simulink model "TestBench_DSD"  (R2021a)
settings: Solver=VariableStepAuto  StartTime=0.0  StopTime=0.05  FixedStep=1e-10  MaxStep=1e-4  RelTol=1e-3
PreLoadFcn:
  | clear;
  | dead_time= 5e-7;
  | T_sample = 1e-7;
  | f_pwm= 8e3;
  | f_el=200;
  | amplitude=0.1;
  | U_dc=800;
  | Iq_soll=200;
  | 
  | load('busdef.mat')
  | 
  | %**** Controller ****
  | L_filter = 70e-6;
  | R_losses = 1.74e-3;
  | PGain = L_filter*0.05*2*pi;
  | IGain = R_losses*0.05*2*pi;
  | 
  | %**** Deadtime Correction ****
  | Rds_on_module = 0.045/15;
  | 
  | %**** Filter ****
  | FilterQuality = 0.7071
InitFcn:
  | %%PGain = (L_filter*0.09*2*pi*f_pwm-R_losses)*0.45;
  | %%IGain = PGain*50/1.2; %% 25 = Period for ringing with too hight PGain
  | 
  | %%PGain = L_filter/(2*(1.5/f_pwm));
  | %%IGain  = PGain*R_losses/L_filter;
undefined symbols (not defined in the file): DiscIntNeverNeededParam, haltPwmSi, haltPwmSic, I_abc_sampled
libraries: nesl_utility x18, simulink x17, fl_lib x15, ee_lib x5, spsFirstOrderFilterLib x3, eeTransforms x2, cstextras x1, spsRMSLib x1, simulink_extras x1, spspowerguiLib x1
(part 1 of 3)
settings Model: Creator=Z634594  LastModifiedBy=Z634594
settings SolverCC: ZeroCrossAlgorithm=Adaptive  AlgebraicLoopSolver=TrustRegion
settings DataIOCC: ReturnWorkspaceOutputs=off
settings DebuggingCC: MergeDetectMultiDrivingBlocksExec=none  SFMachineParentedDataDiag=warning  ArithmeticOperatorsInVariantConditions=warning
settings SFSimCC: SimUseLocalCustomCode=off  CustomCodeUndefinedFunction=UseInterfaceOnly
settings RTWCC: RTWUseLocalCustomCode=off
settings CodeAppCC: StateflowObjectComments=on

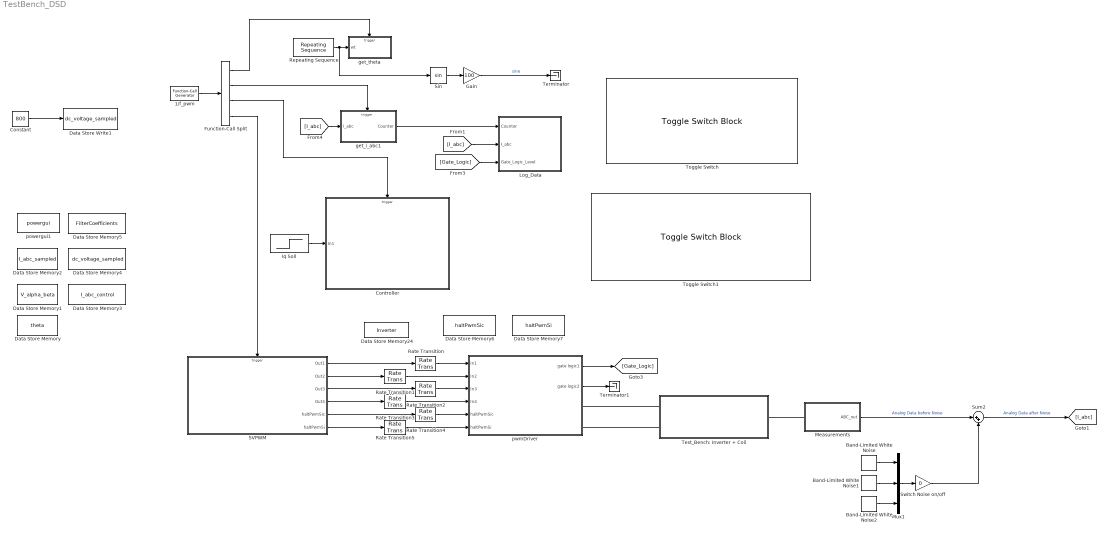
== system TestBench_DSD ==
  1/f_pwm : simulink/Ports & Subsystems/Function-Call Generator  sample_time=1/f_pwm  numberOfIterations=1  DisallowWideOutput=off
  Band-Limited White Noise : simulink/Sources/Band-Limited White Noise  Cov=[0.0004]  Ts=pi/2*1e-6  seed=[40000]
  Band-Limited White Noise1 : simulink/Sources/Band-Limited White Noise  Cov=[0.0004]  Ts=pi/2*1e-6  seed=[35000]
  Band-Limited White Noise2 : simulink/Sources/Band-Limited White Noise  Cov=[0.0004]  Ts=pi/2*1e-6  seed=[30000]
  Constant : Constant  Value=800
  Controller : Subsystem  TreatAsAtomicUnit=on
  Data Store Memory : DataStoreMemory  DataStoreName=theta  ReadBeforeWriteMsg=warning  WriteAfterWriteMsg=warning  WriteAfterReadMsg=warning  ShowAdditionalParam=off
  Data Store Memory1 : DataStoreMemory  DataStoreName=V_alpha_beta  ReadBeforeWriteMsg=warning  WriteAfterWriteMsg=warning  WriteAfterReadMsg=warning  InitialValue=[0 0]  ShowAdditionalParam=off
  Data Store Memory2 : DataStoreMemory  DataStoreName=I_abc_sampled  ReadBeforeWriteMsg=warning  WriteAfterWriteMsg=warning  WriteAfterReadMsg=warning  InitialValue=[0 0 0]  ShowAdditionalParam=off
  Data Store Memory24 : DataStoreMemory  DataStoreName=Inverter  ReadBeforeWriteMsg=warning  WriteAfterWriteMsg=warning  WriteAfterReadMsg=warning  InitialValue=Device_MATLABStruct  ShowAdditionalParam=off  OutDataTypeStr=Bus: Device
  Data Store Memory3 : DataStoreMemory  DataStoreName=I_abc_control  ReadBeforeWriteMsg=warning  WriteAfterWriteMsg=warning  WriteAfterReadMsg=warning  InitialValue=[0 0 0]  ShowAdditionalParam=off
  Data Store Memory4 : DataStoreMemory  DataStoreName=dc_voltage_sampled  ReadBeforeWriteMsg=warning  WriteAfterWriteMsg=warning  WriteAfterReadMsg=warning  InitialValue=U_dc  ShowAdditionalParam=off
  Data Store Memory5 : DataStoreMemory  DataStoreName=FilterCoefficients  ReadBeforeWriteMsg=warning  WriteAfterWriteMsg=warning  WriteAfterReadMsg=warning  InitialValue=[1 0 0 0 0]  ShowAdditionalParam=off
  Data Store Memory6 : DataStoreMemory  DataStoreName=haltPwmSic  ReadBeforeWriteMsg=warning  WriteAfterWriteMsg=warning  WriteAfterReadMsg=warning  InitialValue=[1 1 1]  ShowAdditionalParam=off
  Data Store Memory7 : DataStoreMemory  DataStoreName=haltPwmSi  ReadBeforeWriteMsg=warning  WriteAfterWriteMsg=warning  WriteAfterReadMsg=warning  InitialValue=[0 0 0]  ShowAdditionalParam=off
  Data Store Write1 : DataStoreWrite  DataStoreName=dc_voltage_sampled  IndexOptions=Index vector (dialog)  Indices=1  OutputSizes=1
  Function-Call Split : FunctionCallSplit  IconShape=distinctive  NumOutputPorts=4  OutputPortLayout=default
  Gain : Gain  Gain=100
  Iq Soll : Step  Time=2/f_pwm  After=Iq_soll  SampleTime=0
  Log_Data : Subsystem
  Measurements : Subsystem
  Mux1 : Mux  Inputs=3
  Rate Transition{,1..5} (6 alike) : RateTransition
  Repeating Sequence : simulink/Sources/Repeating Sequence  rep_seq_t=[0 1/f_el]  rep_seq_y=[0 2*pi]
  SVPWM : Subsystem
  Sin : Trigonometry
  Sum2 : Sum  Inputs=|++
  Switch Noise on/off : Gain  Gain=0
  Terminator : Terminator
  Terminator1 : Terminator
  Test_Bench: Inverter + Coil : Subsystem
  Toggle Switch : ToggleSwitchBlock
      settings: Values={{'Off', 'On'}, [0 1]}
  Toggle Switch1 : ToggleSwitchBlock
      settings: Values={{'Off', 'On'}, [0 1]}
  get_i_abc1 : Subsystem  TreatAsAtomicUnit=on
  get_theta : Subsystem  TreatAsAtomicUnit=on
  powergui1 : spspowerguiLib/powergui  Priority=1  SimulationMode=Continuous  SampleTime=1e-9  frequency=60  Iterations=50  frequencyindice=0  Pbase=100e6  ErrMax=1e-4  UnitsV=kV  UnitsW=MW  buscounter=0  FunctionMessages=off  echomessages=off  EnableUseOfTLC=off  CurrentSourceSwitches=off  DisableSnubberDevices=off  DisableRonSwitches=off  DisableVfSwitches=off  DisplayEquations=off  AutomaticDiscreteSolvers=off  SolverType=Tustin/Backward Euler (TBE)  Interpol=off  ExternalGateDelay=off  methode=off  Ts=100  x0status=blocks  SPID=on  SwTol=0  HookPort=off  NonlinearTolerance=1e-4  nMaxIteration=100  ContinueOnMaxIteration=off  RestoreLinks=warning  ResistiveCurrentMeasurement=off  Frange=[0:2:500]  Ylog=off  Xlog=on  ShowGrid=off  save=off  variable=ZData  structure=logsout  ZoomFFT=off  StartTime=0.01  cycles=10  DisplayStyle=1  fundamental=200  FreqAxis=off  MaxFrequency=10000  frequencyindicesteady=1  RmsSteady=1  display=off
  pwmDriver : Subsystem
  wires:
  Repeating Sequence/1 -> Sin/1, get_theta/1(wt)
  [I_abc] -> Log_Data/2(I_abc)
  [Gate_Logic] -> Log_Data/3(Gate_Logic_Level)
  Sum2/1 -> [I_abc]  "Analog Data after Noise"
  Band-Limited White Noise1/1 -> Mux1/2
  Band-Limited White Noise/1 -> Mux1/1
  Band-Limited White Noise2/1 -> Mux1/3
  Mux1/1 -> Switch Noise on/off/1
  Measurements/1(ABC_out) -> Sum2/1  "Analog Data before Noise"
  Switch Noise on/off/1 -> Sum2/2
  Constant/1 -> Data Store Write1/1
  get_i_abc1/1(Counter) -> Log_Data/1(Counter)
  pwmDriver/1(gate logic1) -> [Gate_Logic]
  [I_abc] -> get_i_abc1/1(I_abc)
  1/f_pwm/1 -> Function-Call Split/1
  Function-Call Split/1 -> get_theta/Trigger
  Function-Call Split/2 -> get_i_abc1/Trigger
  Function-Call Split/3 -> Controller/Trigger
  Iq Soll/1 -> Controller/1(In1)
  Function-Call Split/4 -> SVPWM/Trigger
  SVPWM/4(Out4) -> Rate Transition3/1
  SVPWM/3(Out3) -> Rate Transition2/1
  SVPWM/2(Out2) -> Rate Transition1/1
  SVPWM/1(Out1) -> Rate Transition/1
  Rate Transition/1 -> pwmDriver/1(In1)
  Rate Transition1/1 -> pwmDriver/2(In2)
  Rate Transition2/1 -> pwmDriver/3(In3)
  Rate Transition3/1 -> pwmDriver/4(In4)
  Rate Transition4/1 -> pwmDriver/5(haltPwmSic)
  SVPWM/5(haltPwmSic) -> Rate Transition4/1
  SVPWM/6(haltPwmSi) -> Rate Transition5/1
  Rate Transition5/1 -> pwmDriver/6(haltPwmSi)
  Sin/1 -> Gain/1
  Gain/1 -> Terminator/1  "sine"
  pwmDriver/2(gate logic2) -> Terminator1/1
  connections:
  Test_Bench: Inverter + Coil/LConn1 -- pwmDriver/RConn1
  Measurements/LConn1 -- Test_Bench: Inverter + Coil/RConn1
  Test_Bench: Inverter + Coil/LConn2 -- pwmDriver/RConn2

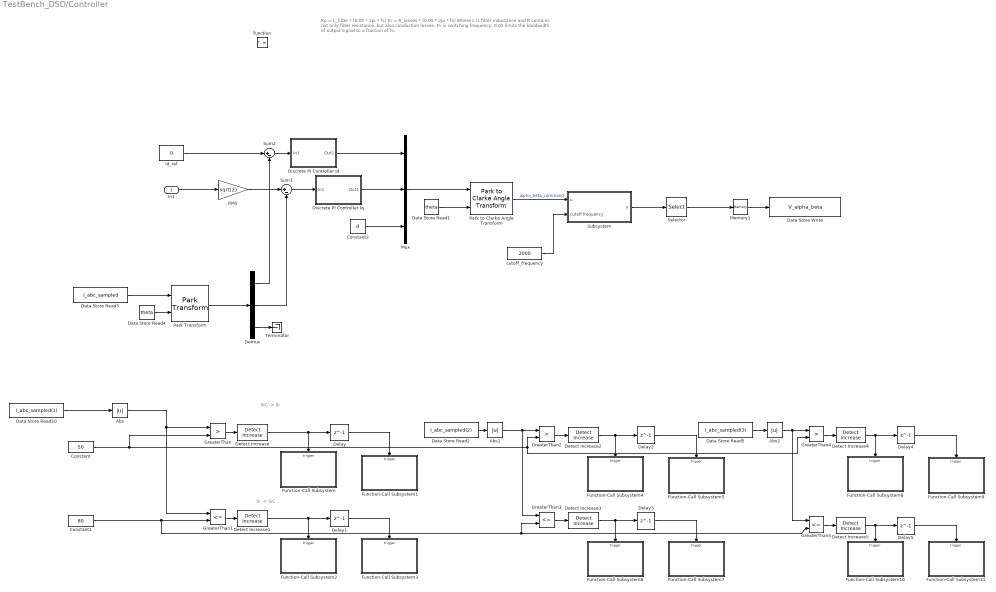
== system TestBench_DSD/Controller ==
  note: Kp = L_filter * (0.05 * 2pi * fs)
      |
      | Ki = R_losses * (0.05 * 2pi * fs)
      |
      | Where L is filter inductance and R contains not only filter resistance, but also conduction losses.
      | Fs is switching frequency.
      | 0.05 limits the bandwidth of output signal to a fraction of fs.
  note: Si -> SiC
  note: SiC -> Si
  In1 : Inport
  function : TriggerPort  TriggerType=function-call  VariantControl=Variant
  Abs : Abs
  Abs1 : Abs
  Abs2 : Abs
  Constant : Constant  Value=50
  Constant1 : Constant  Value=80
  Constant2 : Constant  Value=0
  Data Store Read1 : DataStoreRead  DataStoreName=theta  IndexOptions=Index vector (dialog)  Indices=1  OutputSizes=1
  Data Store Read10 : DataStoreRead  DataStoreName=I_abc_sampled  DataStoreElements=I_abc_sampled(1)  IndexOptions=Index vector (dialog)  Indices=1  OutputSizes=1
  Data Store Read2 : DataStoreRead  DataStoreName=I_abc_sampled  DataStoreElements=I_abc_sampled(2)  IndexOptions=Index vector (dialog)  Indices=1  OutputSizes=1
  Data Store Read3 : DataStoreRead  DataStoreName=I_abc_sampled  IndexOptions=Index vector (dialog)  Indices=1  OutputSizes=1
  Data Store Read4 : DataStoreRead  DataStoreName=theta  IndexOptions=Index vector (dialog)  Indices=1  OutputSizes=1
  Data Store Read5 : DataStoreRead  DataStoreName=I_abc_sampled  DataStoreElements=I_abc_sampled(3)  IndexOptions=Index vector (dialog)  Indices=1  OutputSizes=1
  Data Store Write : DataStoreWrite  DataStoreName=V_alpha_beta  IndexOptions=Index vector (dialog)  Indices=1  OutputSizes=1
  Delay{,1..5} (6 alike) : Delay  DelayLength=1
  Demux : Demux  Outputs=3
  Detect Increase{,1..5} (6 alike) : simulink/Logic and Bit Operations/Detect Increase  vinit=0.0  OutDataTypeStr=boolean
  Discrete PI Controller Id : Subsystem
  Discrete PI Controller Iq : Subsystem
  Function-Call Subsystem : Subsystem  TreatAsAtomicUnit=on
  Function-Call Subsystem1 : Subsystem  TreatAsAtomicUnit=on
  Function-Call Subsystem10 : Subsystem  TreatAsAtomicUnit=on
  Function-Call Subsystem11 : Subsystem  TreatAsAtomicUnit=on
  Function-Call Subsystem2 : Subsystem  TreatAsAtomicUnit=on
  Function-Call Subsystem3 : Subsystem  TreatAsAtomicUnit=on
  Function-Call Subsystem4 : Subsystem  TreatAsAtomicUnit=on
  Function-Call Subsystem5 : Subsystem  TreatAsAtomicUnit=on
  Function-Call Subsystem6 : Subsystem  TreatAsAtomicUnit=on
  Function-Call Subsystem7 : Subsystem  TreatAsAtomicUnit=on
  Function-Call Subsystem8 : Subsystem  TreatAsAtomicUnit=on
  Function-Call Subsystem9 : Subsystem  TreatAsAtomicUnit=on
  GreaterThan : RelationalOperator  Operator=>  OutDataTypeStr=boolean  RndMeth=Simplest
  GreaterThan1 : RelationalOperator  Operator=<=  OutDataTypeStr=boolean  RndMeth=Simplest
  GreaterThan2 : RelationalOperator  Operator=>  OutDataTypeStr=boolean  RndMeth=Simplest
  GreaterThan3 : RelationalOperator  Operator=<=  OutDataTypeStr=boolean  RndMeth=Simplest
  GreaterThan4 : RelationalOperator  Operator=>  OutDataTypeStr=boolean  RndMeth=Simplest
  GreaterThan5 : RelationalOperator  Operator=<=  OutDataTypeStr=boolean  RndMeth=Simplest
  Id_ref : Constant  Value=0
  Memory1 : Memory  InheritSampleTime=on  LinearizeAsDelay=on
  Mux : Mux  Inputs=3
  Park Transform : eeTransforms/Park Transform  AxisAlignment=Q-axis  PowerInvariant=off
  Park to Clarke Angle Transform : eeTransforms/Park to Clarke Angle Transform  AxisAlignment=Q-axis
      settings: SourceProductBaseCode=PS
  RMS : Gain  Gain=sqrt(2)
  Selector : Selector  InputPortWidth=3  IndexOptions=Index vector (dialog)  Indices=[1 2]  OutputSizes=1
  Subsystem : Subsystem
  Sum1 : Sum  Inputs=|+-
  Sum2 : Sum  Inputs=|+-
  Terminator : Terminator
  cutoff_frequency : Constant  Value=2000
  wires:
  Demux/1 -> Sum2/2
  Mux/1 -> Park to Clarke Angle Transform/1
  Demux/3 -> Terminator/1
  Demux/2 -> Sum1/2
  Constant2/1 -> Mux/3
  Sum2/1 -> Discrete PI Controller Id/1(In1)
  Sum1/1 -> Discrete PI Controller Iq/1(In1)
  Discrete PI Controller Iq/1(Out1) -> Mux/2
  Data Store Read3/1 -> Park Transform/1
  Data Store Read4/1 -> Park Transform/2
  Data Store Read1/1 -> Park to Clarke Angle Transform/2
  Memory1/1 -> Data Store Write/1
  Discrete PI Controller Id/1(Out1) -> Mux/1
  Park Transform/1 -> Demux/1
  Selector/1 -> Memory1/1
  Id_ref/1 -> Sum2/1
  In1/1 -> RMS/1
  RMS/1 -> Sum1/1
  cutoff_frequency/1 -> Subsystem/2(cutoff frequency)
  Park to Clarke Angle Transform/1 -> Subsystem/1(u)  "alpha_beta_command"
  Subsystem/1(y) -> Selector/1
  Delay1/1 -> Function-Call Subsystem3/Trigger
  Delay/1 -> Function-Call Subsystem1/Trigger
  Delay2/1 -> Function-Call Subsystem5/Trigger
  Delay5/1 -> Function-Call Subsystem11/Trigger
  Delay4/1 -> Function-Call Subsystem9/Trigger
  GreaterThan1/1 -> Detect Increase1/1
  Delay3/1 -> Function-Call Subsystem7/Trigger
  GreaterThan/1 -> Detect Increase/1
  Data Store Read10/1 -> Abs/1
  Abs/1 -> GreaterThan1/1, GreaterThan/1
  Data Store Read2/1 -> Abs1/1
  Abs1/1 -> GreaterThan3/1, GreaterThan2/1
  GreaterThan2/1 -> Detect Increase2/1
  GreaterThan3/1 -> Detect Increase3/1
  Data Store Read5/1 -> Abs2/1
  Abs2/1 -> GreaterThan5/1, GreaterThan4/1
  Constant/1 -> GreaterThan/2, GreaterThan4/2, GreaterThan2/2
  Constant1/1 -> GreaterThan5/2, GreaterThan3/2, GreaterThan1/2
  Detect Increase/1 -> Delay/1, Function-Call Subsystem/Trigger
  Detect Increase1/1 -> Delay1/1, Function-Call Subsystem2/Trigger
  Detect Increase2/1 -> Function-Call Subsystem4/Trigger, Delay2/1
  Detect Increase3/1 -> Function-Call Subsystem6/Trigger, Delay3/1
  GreaterThan4/1 -> Detect Increase4/1
  Detect Increase4/1 -> Function-Call Subsystem8/Trigger, Delay4/1
  GreaterThan5/1 -> Detect Increase5/1
  Detect Increase5/1 -> Function-Call Subsystem10/Trigger, Delay5/1

== system TestBench_DSD/Log_Data ==
  Counter : Inport
  I_abc : Inport  Port=2
  Gate_Logic_Level : Inport  Port=3
  Data Store Read1 : DataStoreRead  DataStoreName=I_abc_sampled  IndexOptions=Index vector (dialog)  Indices=1  OutputSizes=1
  Data Store Read2 : DataStoreRead  DataStoreName=I_abc_control  IndexOptions=Index vector (dialog)  Indices=1  OutputSizes=1
  Delay : Delay  DelayLength=1  SampleTime=T_sample
  Gain : Gain  Gain=50
  Logical Operator : Logic  Operator=XOR  AllPortsSameDT=off  OutDataTypeStr=boolean
  Product : Product
  Scope1 : Scope  NumInputPorts=3
  Scope6 : Scope  NumInputPorts=5
  wires:
  Delay/1 -> Scope1/2, Logical Operator/1
  Data Store Read1/1 -> Product/2, Scope6/1
  Counter/1 -> Scope1/1, Logical Operator/2, Delay/1
  Product/1 -> Scope6/3
  Logical Operator/1 -> Scope1/3, Product/1
  Gain/1 -> Scope6/4
  I_abc/1 -> Scope6/2
  Gate_Logic_Level/1 -> Gain/1
  Data Store Read2/1 -> Scope6/5

== system TestBench_DSD/Measurements ==
  First-Order Filter : spsFirstOrderFilterLib/First-Order Filter  FilterType=Lowpass  Tc=25e-6  Ts=0  Initialize=off  Vac_Init=[0, 0, 60]  Vdc_Init=0  PlotResponse=off  FreqRange="[0,  200,  1]"
  PS-Simulink Converter1 : nesl_utility/PS-Simulink Converter  PhysicalDomain=network_engine_domain  SubClassName=ps_output  LeftPortType=input  RightPortType=output  PseudoPeriodic=off  Frequencies=[]  Unit=1  AffineConversion=off
      settings: SourceProductBaseCode=PW,SS
  RMS : spsRMSLib/RMS  TrueRMS=on  Freq=f_el  RMSInit=0  Ts=0
  Terminator : Terminator
  Terminator1 : Terminator
  ABC_in : PMIOPort  Side=Left
  ABC_out : Outport  VectorParamsAs1DForOutWhenUnconnected=off
  wires:
  PS-Simulink Converter1/1 -> RMS/1, First-Order Filter/1, ABC_out/1
  RMS/1 -> Terminator/1  "rmsCurrent3Phase"
  First-Order Filter/1 -> Terminator1/1  "phaseCurrent3Phase"
  connections:
  PS-Simulink Converter1/LConn1 -- ABC_in/RConn1

== system TestBench_DSD/SVPWM ==
  function : TriggerPort  TriggerType=function-call  VariantControl=(inherit)
  Data Store Read : DataStoreRead  DataStoreName=V_alpha_beta  IndexOptions=Index vector (dialog)  Indices=1  OutputSizes=1
  Data Store Read1 : DataStoreRead  DataStoreName=I_abc_sampled  IndexOptions=Index vector (dialog)  Indices=1  OutputSizes=1
  Data Store Read2 : DataStoreRead  DataStoreName=dc_voltage_sampled  IndexOptions=Index vector (dialog)  Indices=1  OutputSizes=1
  Data Store Read5 : DataStoreRead  DataStoreName=dc_voltage_sampled  IndexOptions=Index vector (dialog)  Indices=1  OutputSizes=1
  Demux : Demux  Outputs=2
  Divide : Product  Inputs=*/
  Gate_Signal_Voltage1 : Subsystem
  Model : ModelReference  ModelNameDialog=sort_dutycycles.slx  SimulationMode=Normal  ModelReferenceVersion=1.5
  SVPWM : Subsystem
  Terminator : Terminator
  Out1 : Outport
  Out2 : Outport  Port=2
  Out3 : Outport  Port=3
  Out4 : Outport  Port=4
  haltPwmSic : Outport  Port=5
  haltPwmSi : Outport  Port=6
  wires:
  Divide/1 -> Demux/1
  Data Store Read5/1 -> Divide/2
  SVPWM/1(Sector Number) -> Model/1
  SVPWM/2(Ta Tb T0 normalized) -> Model/2
  Data Store Read/1 -> Divide/1
  Demux/2 -> SVPWM/2(U_angle)
  Model/2 -> Terminator/1
  Demux/1 -> SVPWM/1(U_mag)
  Model/1 -> Gate_Signal_Voltage1/1(dutycycles)  "Duty Cycles Rearranged"
  Data Store Read1/1 -> Gate_Signal_Voltage1/2(phaseCurrent)
  Gate_Signal_Voltage1/2(Out2) -> Out2/1
  Gate_Signal_Voltage1/4(Out4) -> Out4/1
  Gate_Signal_Voltage1/3(Out3) -> Out3/1
  Gate_Signal_Voltage1/1(Out1) -> Out1/1
  Gate_Signal_Voltage1/5(haltPwmSic) -> haltPwmSic/1
  Gate_Signal_Voltage1/6(haltPwmSi) -> haltPwmSi/1
  Data Store Read2/1 -> Gate_Signal_Voltage1/3(dcLinkVoltage)

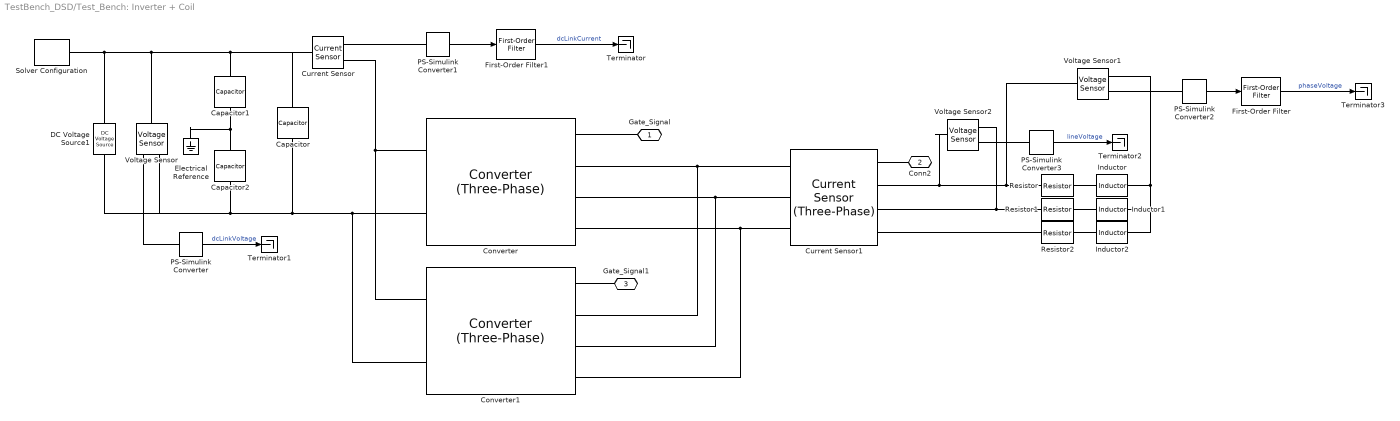
== system TestBench_DSD/Test_Bench: Inverter + Coil ==
  Capacitor : fl_lib/Electrical/Electrical Elements/Capacitor  c=550e-6 F  r=1e-6 Ohm  g=0 1/Ohm  i_specify=off  i_priority=None  i=0 A  i_nominal_specify=off  i_nominal_unit=A  i_nominal_value=1  v_specify=off  v_priority=None  v=0 V  v_nominal_specify=off  v_nominal_unit=V  v_nominal_value=1  vc_specify=on  vc_priority=High  vc=U_dc V  vc_nominal_specify=off  vc_nominal_unit=V  vc_nominal_value=1
  Capacitor1 : fl_lib/Electrical/Electrical Elements/Capacitor  c=100e-9 F  r=1e-6 Ohm  g=0 1/Ohm  i_specify=off  i_priority=None  i=0 A  i_nominal_specify=off  i_nominal_unit=A  i_nominal_value=1  v_specify=off  v_priority=None  v=0 V  v_nominal_specify=off  v_nominal_unit=V  v_nominal_value=1  vc_specify=on  vc_priority=High  vc=U_dc/2 V  vc_nominal_specify=off  vc_nominal_unit=V  vc_nominal_value=1
  Capacitor2 : fl_lib/Electrical/Electrical Elements/Capacitor  c=100e-9 F  r=1e-6 Ohm  g=0 1/Ohm  i_specify=off  i_priority=None  i=0 A  i_nominal_specify=off  i_nominal_unit=A  i_nominal_value=1  v_specify=off  v_priority=None  v=0 V  v_nominal_specify=off  v_nominal_unit=V  v_nominal_value=1  vc_specify=on  vc_priority=High  vc=U_dc/2 V  vc_nominal_specify=off  vc_nominal_unit=V  vc_nominal_value=1
  Converter : ee_lib/Semiconductors & Converters/Converters/Converter (Three-Phase)  device_type=ee.enum.converters.switchingdevice.mosfet  Vf=0.8 V  Ron=0.001 Ohm  Rds=Rds_on_module Ohm  Goff=1e-9 1/Ohm  Vth=4 V  Vgt=1 V  Vgt_off=-1 V  Ih=1 A  diode_param=ee.enum.converters.protectiondiode.nodynamics  diode_Vf=2 V  diode_Ron=Rds_on_module Ohm  diode_Goff=1e-9 1/Ohm  diode_C=50 nF  diode_iRM=-235 A  diode_iF=300 A  diode_idot=-50 A/us  diode_trr_param=ee.enum.converters.diodetrr.trr_factor  diode_trr_factor=3  diode_trr=15 us  diode_Qrr=1.5e+3 s*uA  snubber_type=ee.enum.converters.snubber.exclude  Rs=0.01 Ohm  Cs=1e-6 F
      settings: SourceProductBaseCode=PS  InternalSimscapePortConfiguration="{\"Bottom\":[],\"Left\":[{\"id\":\"G\",\"label\":\"G\",\"type\":\"foundation.electrical.twelve_phase\"},{\"id\":\"a\",\"label\":\"a\",\"type\":\"foundation.electrical.electrical\"},{\"id\":\"b\",\"label\":\"b\",\"type\":\"foundation.electrical.electrical\"},{\"id\":\"c\",\"label\":\"c\",\"type\":\"foundation.electrical.electrical\"}],\"Right\":[{\"id\":\"p\",\"label\":\"+\",\"type\":\"foundation.electrical.electrical\"},{\"id\":\"n\",\"label\":\"-\",\"type\":\"foundation.electrical.electrical\"}],\"Top\":[]}"
  Converter1 : ee_lib/Semiconductors & Converters/Converters/Converter (Three-Phase)  device_type=ee.enum.converters.switchingdevice.igbt  Vf=0.8 V  Ron=0.001 Ohm  Rds=Rds_on_module Ohm  Goff=1e-9 1/Ohm  Vth=4 V  Vgt=1 V  Vgt_off=-1 V  Ih=1 A  diode_param=ee.enum.converters.protectiondiode.nodynamics  diode_Vf=0.8 V  diode_Ron=0.001 Ohm  diode_Goff=1e-9 1/Ohm  diode_C=50 nF  diode_iRM=-235 A  diode_iF=300 A  diode_idot=-50 A/us  diode_trr_param=ee.enum.converters.diodetrr.trr_factor  diode_trr_factor=3  diode_trr=15 us  diode_Qrr=1.5e+3 s*uA  snubber_type=ee.enum.converters.snubber.exclude  Rs=0.01 Ohm  Cs=1e-6 F
      settings: SourceProductBaseCode=PS  InternalSimscapePortConfiguration="{\"Bottom\":[],\"Left\":[{\"id\":\"G\",\"label\":\"G\",\"type\":\"foundation.electrical.twelve_phase\"},{\"id\":\"a\",\"label\":\"a\",\"type\":\"foundation.electrical.electrical\"},{\"id\":\"b\",\"label\":\"b\",\"type\":\"foundation.electrical.electrical\"},{\"id\":\"c\",\"label\":\"c\",\"type\":\"foundation.electrical.electrical\"}],\"Right\":[{\"id\":\"p\",\"label\":\"+\",\"type\":\"foundation.electrical.electrical\"},{\"id\":\"n\",\"label\":\"-\",\"type\":\"foundation.electrical.electrical\"}],\"Top\":[]}"
  Current Sensor : fl_lib/Electrical/Electrical Sensors/Current Sensor
  Current Sensor1 : ee_lib/Sensors & Transducers/Current Sensor (Three-Phase)
      settings: InternalSimscapePortConfiguration="{\"Bottom\":[],\"Left\":[{\"id\":\"a1\",\"label\":\"a1\",\"type\":\"foundation.electrical.electrical\"},{\"id\":\"b1\",\"label\":\"b1\",\"type\":\"foundation.electrical.electrical\"},{\"id\":\"c1\",\"label\":\"c1\",\"type\":\"foundation.electrical.electrical\"}],\"Right\":[{\"id\":\"I_output\",\"label\":\"I\",\"type\":\"output\"},{\"id\":\"a2\",\"label\":\"a2\",\"type\":\"foundation.electrical.electrical\"},{\"id\":\"b2\",\"label\":\"b2\",\"type\":\"foundation.electrical.electrical\"},{\"id\":\"c2\",\"label\":\"c2\",\"type\":\"foundation.electrical.electrical\"}],\"Top\":[]}"
  DC Voltage Source1 : fl_lib/Electrical/Electrical Sources/DC Voltage Source  v0=U_dc V
  Electrical Reference : fl_lib/Electrical/Electrical Elements/Electrical Reference
  First-Order Filter : spsFirstOrderFilterLib/First-Order Filter  FilterType=Lowpass  Tc=250e-6  Ts=0  Initialize=off  Vac_Init=[0, 0, 60]  Vdc_Init=0  PlotResponse=off  FreqRange="[0,  200,  1]"
  First-Order Filter1 : spsFirstOrderFilterLib/First-Order Filter  FilterType=Lowpass  Tc=100e-6  Ts=0  Initialize=off  Vac_Init=[0, 0, 60]  Vdc_Init=0  PlotResponse=off  FreqRange="[0,  200,  1]"
  Inductor : fl_lib/Electrical/Electrical Elements/Inductor  l=70e-6 H  r=0 Ohm  g=1e-9 1/Ohm  i_specify=off  i_priority=None  i=0 A  i_nominal_specify=off  i_nominal_unit=A  i_nominal_value=1  v_specify=off  v_priority=None  v=0 V  v_nominal_specify=off  v_nominal_unit=V  v_nominal_value=1  i_L_specify=off  i_L_priority=High  i_L=0 A  i_L_nominal_specify=off  i_L_nominal_unit=A  i_L_nominal_value=1
  Inductor1 : fl_lib/Electrical/Electrical Elements/Inductor  l=70e-6 H  r=0 Ohm  g=1e-9 1/Ohm  i_specify=off  i_priority=None  i=0 A  i_nominal_specify=off  i_nominal_unit=A  i_nominal_value=1  v_specify=off  v_priority=None  v=0 V  v_nominal_specify=off  v_nominal_unit=V  v_nominal_value=1  i_L_specify=off  i_L_priority=High  i_L=0 A  i_L_nominal_specify=off  i_L_nominal_unit=A  i_L_nominal_value=1
  Inductor2 : fl_lib/Electrical/Electrical Elements/Inductor  l=70e-6 H  r=0 Ohm  g=1e-9 1/Ohm  i_specify=off  i_priority=None  i=0 A  i_nominal_specify=off  i_nominal_unit=A  i_nominal_value=1  v_specify=off  v_priority=None  v=0 V  v_nominal_specify=off  v_nominal_unit=V  v_nominal_value=1  i_L_specify=off  i_L_priority=High  i_L=0 A  i_L_nominal_specify=off  i_L_nominal_unit=A  i_L_nominal_value=1
  PS-Simulink Converter{,1..3} (4 alike) : nesl_utility/PS-Simulink Converter  PhysicalDomain=network_engine_domain  SubClassName=ps_output  LeftPortType=input  RightPortType=output  PseudoPeriodic=off  Frequencies=[]  Unit=1  AffineConversion=off
      settings: SourceProductBaseCode=PW,SS
  Resistor : fl_lib/Electrical/Electrical Elements/Resistor  R=1.74e-3 Ohm  i_specify=off  i_priority=None  i=0 A  i_nominal_specify=off  i_nominal_unit=A  i_nominal_value=1  v_specify=off  v_priority=None  v=0 V  v_nominal_specify=off  v_nominal_unit=V  v_nominal_value=1
  Resistor1 : fl_lib/Electrical/Electrical Elements/Resistor  R=1.74e-3 Ohm  i_specify=off  i_priority=None  i=0 A  i_nominal_specify=off  i_nominal_unit=A  i_nominal_value=1  v_specify=off  v_priority=None  v=0 V  v_nominal_specify=off  v_nominal_unit=V  v_nominal_value=1
  Resistor2 : fl_lib/Electrical/Electrical Elements/Resistor  R=1.74e-3 Ohm  i_specify=off  i_priority=None  i=0 A  i_nominal_specify=off  i_nominal_unit=A  i_nominal_value=1  v_specify=off  v_priority=None  v=0 V  v_nominal_specify=off  v_nominal_unit=V  v_nominal_value=1
  Solver Configuration : nesl_utility/Solver Configuration  PhysicalDomain=network_engine_domain  SubClassName=solver  LeftPortType=input  RightPortType=generic  Tones=[]  Harmonics=[]  SimulateNoise=off  Profile=off  UseLocalSampling=off  EnableSwitchedLinearOptims=on  FrequencyDomain=off  UseCCode=off  RelTol=0.001  AbsTol=1e-06  MinStep=1e-09  ToWorkspace=off  RevertToSquareIcSolve=off  NumHomotopyIterations=100  PhasorMode=off  PhasorModeNumHarmonics=1  DoDC=off  ResidualTolerance=1e-09  UseLocalSolver=off  LocalSolverChoice=NE_BACKWARD_EULER_ADVANCER  LocalSolverSampleTime=0.001  DoFixedCost=off  MaxNonlinIter=3  MaxModeIter=2  ComputeImpulses=off  ImpulseIterations=2  LinearAlgebra=Sparse  EquationFormulation=NE_TIME_EF  DelaysMemoryBudget=1024  AutomaticFiltering=on  FilteringTimeConstant=0.001  PartitionStorageMethod=AS_NEEDED  PartitionMemoryBudget=1024  PartitionMethod=FAST
      settings: SourceProductBaseCode=PW,SS
  Terminator{,1..3} (4 alike) : Terminator
  Voltage Sensor : fl_lib/Electrical/Electrical Sensors/Voltage Sensor
  Voltage Sensor1 : fl_lib/Electrical/Electrical Sensors/Voltage Sensor
  Voltage Sensor2 : fl_lib/Electrical/Electrical Sensors/Voltage Sensor
  Gate_Signal : PMIOPort  Side=Left
  Conn2 : PMIOPort  Port=2  Side=Right
  Gate_Signal1 : PMIOPort  Port=3  Side=Left
  wires:
  First-Order Filter1/1 -> Terminator/1  "dcLinkCurrent"
  PS-Simulink Converter/1 -> Terminator1/1  "dcLinkVoltage"
  PS-Simulink Converter1/1 -> First-Order Filter1/1
  PS-Simulink Converter2/1 -> First-Order Filter/1
  PS-Simulink Converter3/1 -> Terminator2/1  "lineVoltage"
  First-Order Filter/1 -> Terminator3/1  "phaseVoltage"
  connections:
  Voltage Sensor1/RConn2 -- Inductor2/RConn1 -- Inductor1/RConn1 -- Inductor/RConn1
  Current Sensor1/LConn1 -- Converter1/LConn2 -- Converter/LConn2
  Current Sensor1/LConn2 -- Converter1/LConn3 -- Converter/LConn3
  Current Sensor1/RConn2 -- Resistor/LConn1 -- Voltage Sensor1/LConn1 -- Voltage Sensor2/LConn1
  Resistor/RConn1 -- Inductor/LConn1
  Converter/LConn1 -- Gate_Signal/RConn1
  Resistor1/RConn1 -- Inductor1/LConn1
  Current Sensor1/RConn4 -- Resistor2/LConn1
  Current Sensor1/RConn3 -- Resistor1/LConn1 -- Voltage Sensor2/RConn2
  Resistor2/RConn1 -- Inductor2/LConn1
  Current Sensor1/LConn3 -- Converter1/LConn4 -- Converter/LConn4
  Capacitor/RConn1 -- Capacitor2/RConn1 -- DC Voltage Source1/RConn1 -- Voltage Sensor/RConn2 -- Converter1/RConn2 -- Converter/RConn2
  Current Sensor/RConn2 -- Converter1/RConn1 -- Converter/RConn1
  PS-Simulink Converter/LConn1 -- Voltage Sensor/RConn1
  PS-Simulink Converter1/LConn1 -- Current Sensor/RConn1
  Voltage Sensor/LConn1 -- Capacitor1/LConn1 -- Capacitor/LConn1 -- Current Sensor/LConn1 -- DC Voltage Source1/LConn1 -- Solver Configuration/RConn1
  Conn2/RConn1 -- Current Sensor1/RConn1
  PS-Simulink Converter2/LConn1 -- Voltage Sensor1/RConn1
  PS-Simulink Converter3/LConn1 -- Voltage Sensor2/RConn1
  Capacitor2/LConn1 -- Electrical Reference/LConn1 -- Capacitor1/RConn1
  Gate_Signal1/RConn1 -- Converter1/LConn1

== system TestBench_DSD/get_i_abc1 ==
  note: Digital Biquad Filter (IIR)
      | Transposed Direct Form 2
  I_abc : Inport
  function : TriggerPort  TriggerType=function-call  VariantControl=Variant
  Counter Limited : simulink/Sources/Counter Limited  uplimit=1  tsamp=-1
  Data Store Write : DataStoreWrite  DataStoreName=I_abc_sampled  IndexOptions=Index vector (dialog)  Indices=1  OutputSizes=1
  Delay1 : Delay  DelayLength=1
  Delay3 : Delay  DelayLength=1
  Gain : Gain  Gain=0.13491016791740667
  Gain1 : Gain  Gain=-1.1429772843080923
  Gain2 : Gain  Gain=0.41279762014290533
  Gain3 : Gain  Gain=0.06745508395870334
  Gain4 : Gain  Gain=0.06745508395870334
  Scope : Scope  NumInputPorts=3
  Sum : Sum  Inputs=++-
  Sum1 : Sum  Inputs=+|-
  Sum2 : Sum  Inputs=|++
  Counter : Outport  VectorParamsAs1DForOutWhenUnconnected=off
  wires:
  Counter Limited/1 -> Counter/1
  Gain/1 -> Sum/1
  Gain1/1 -> Sum/3
  Gain3/1 -> Sum1/1
  Gain2/1 -> Sum1/2
  Gain4/1 -> Sum2/1
  Delay1/1 -> Sum2/2
  Sum/1 -> Delay1/1
  Delay3/1 -> Sum/2
  Sum1/1 -> Delay3/1
  Sum2/1 -> Gain2/1, Gain1/1, Scope/1
  I_abc/1 -> Scope/2, Data Store Write/1, Gain4/1, Gain/1, Gain3/1

== system TestBench_DSD/get_theta ==
  wt : Inport
  function : TriggerPort  TriggerType=function-call  VariantControl=Variant
  Data Store Write : DataStoreWrite  DataStoreName=theta  IndexOptions=Index vector (dialog)  Indices=1  OutputSizes=1
  wires:
  wt/1 -> Data Store Write/1

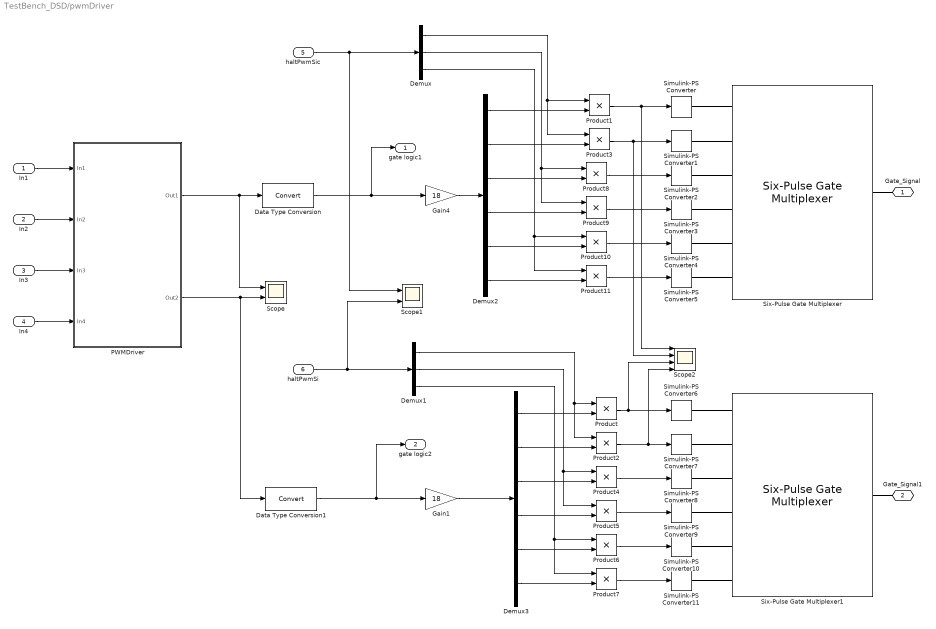
== system TestBench_DSD/pwmDriver ==
  In1 : Inport
  In2 : Inport  Port=2
  In3 : Inport  Port=3
  In4 : Inport  Port=4
  haltPwmSic : Inport  Port=5
  haltPwmSi : Inport  Port=6
  Data Type Conversion : DataTypeConversion
  Data Type Conversion1 : DataTypeConversion
  Demux : Demux  Outputs=3
  Demux1 : Demux  Outputs=3
  Demux2 : Demux  Outputs=6
  Demux3 : Demux  Outputs=6
  Gain1 : Gain  Gain=18
  Gain4 : Gain  Gain=18
  PWMDriver : Subsystem
  Product{,1..11} (12 alike) : Product
  Scope : Scope  NumInputPorts=2
  Scope1 : Scope  NumInputPorts=2
  Scope2 : Scope  NumInputPorts=4
  Simulink-PS Converter{,1..11} (12 alike) : nesl_utility/Simulink-PS Converter  PhysicalDomain=network_engine_domain  SubClassName=ps_input  LeftPortType=input  RightPortType=output  PseudoPeriodic=off  Frequencies=[]  NoiseDistribution=none  NoiseParameters=[]  Unit=1  AffineConversion=off  FilteringAndDerivatives=provide  SimscapeFilterOrder=1  InputFilterTimeConstant=0.001  UdotUserProvided=0
      settings: SourceProductBaseCode=PW,SS
  Six-Pulse Gate Multiplexer : ee_lib/Semiconductors & Converters/Converters/Six-Pulse Gate Multiplexer  R=0 Ohm
      settings: SourceProductBaseCode=PS  InternalSimscapePortConfiguration="{\"Bottom\":[],\"Left\":[{\"id\":\"GaH\",\"label\":\"Ga(H)\",\"type\":\"input\"},{\"id\":\"GaL\",\"label\":\"Ga(L)\",\"type\":\"input\"},{\"id\":\"GbH\",\"label\":\"Gb(H)\",\"type\":\"input\"},{\"id\":\"GbL\",\"label\":\"Gb(L)\",\"type\":\"input\"},{\"id\":\"GcH\",\"label\":\"Gc(H)\",\"type\":\"input\"},{\"id\":\"GcL\",\"label\":\"Gc(L)\",\"type\":\"input\"}],\"Right\":[{\"id\":\"p\",\"label\":\"G\",\"type\":\"foundation.electrical.twelve_phase\"}],\"Top\":[]}"
  Six-Pulse Gate Multiplexer1 : ee_lib/Semiconductors & Converters/Converters/Six-Pulse Gate Multiplexer  R=0 Ohm
      settings: SourceProductBaseCode=PS  InternalSimscapePortConfiguration="{\"Bottom\":[],\"Left\":[{\"id\":\"GaH\",\"label\":\"Ga(H)\",\"type\":\"input\"},{\"id\":\"GaL\",\"label\":\"Ga(L)\",\"type\":\"input\"},{\"id\":\"GbH\",\"label\":\"Gb(H)\",\"type\":\"input\"},{\"id\":\"GbL\",\"label\":\"Gb(L)\",\"type\":\"input\"},{\"id\":\"GcH\",\"label\":\"Gc(H)\",\"type\":\"input\"},{\"id\":\"GcL\",\"label\":\"Gc(L)\",\"type\":\"input\"}],\"Right\":[{\"id\":\"p\",\"label\":\"G\",\"type\":\"foundation.electrical.twelve_phase\"}],\"Top\":[]}"
  Gate_Signal : PMIOPort  Side=Right
  Gate_Signal1 : PMIOPort  Port=2  Side=Right
  gate logic1 : Outport  VectorParamsAs1DForOutWhenUnconnected=off
  gate logic2 : Outport  Port=2  VectorParamsAs1DForOutWhenUnconnected=off
  wires:
  Product5/1 -> Simulink-PS Converter9/1
  In4/1 -> PWMDriver/4(In4)
  Product2/1 -> Scope2/4, Simulink-PS Converter7/1
  PWMDriver/2(Out2) -> Scope/2, Data Type Conversion1/1
  Data Type Conversion/1 -> gate logic1/1, Gain4/1
  Data Type Conversion1/1 -> gate logic2/1, Gain1/1
  Gain1/1 -> Demux3/1
  In2/1 -> PWMDriver/2(In2)
  haltPwmSic/1 -> Scope1/1, Demux/1
  Product3/1 -> Scope2/2, Simulink-PS Converter1/1
  Demux3/6 -> Product7/2
  PWMDriver/1(Out1) -> Data Type Conversion/1, Scope/1
  haltPwmSi/1 -> Demux1/1, Scope1/2
  Demux3/1 -> Product/2
  Demux3/2 -> Product2/2
  Demux2/1 -> Product1/2
  Demux3/3 -> Product4/2
  In3/1 -> PWMDriver/3(In3)
  Demux3/4 -> Product5/2
  Gain4/1 -> Demux2/1
  Product6/1 -> Simulink-PS Converter10/1
  Demux3/5 -> Product6/2
  Product4/1 -> Simulink-PS Converter8/1
  Product7/1 -> Simulink-PS Converter11/1
  Product1/1 -> Scope2/1, Simulink-PS Converter/1
  Demux2/2 -> Product3/2
  Product/1 -> Scope2/3, Simulink-PS Converter6/1
  In1/1 -> PWMDriver/1(In1)
  Demux/1 -> Product3/1, Product1/1
  Product8/1 -> Simulink-PS Converter2/1
  Product9/1 -> Simulink-PS Converter3/1
  Product10/1 -> Simulink-PS Converter4/1
  Product11/1 -> Simulink-PS Converter5/1
  Demux/2 -> Product9/1, Product8/1
  Demux/3 -> Product11/1, Product10/1
  Demux2/3 -> Product8/2
  Demux2/4 -> Product9/2
  Demux2/5 -> Product10/2
  Demux2/6 -> Product11/2
  Demux1/1 -> Product2/1, Product/1
  Demux1/2 -> Product4/1, Product5/1
  Demux1/3 -> Product7/1, Product6/1
  connections:
  Simulink-PS Converter6/RConn1 -- Six-Pulse Gate Multiplexer1/LConn1
  Simulink-PS Converter1/RConn1 -- Six-Pulse Gate Multiplexer/LConn2
  Simulink-PS Converter5/RConn1 -- Six-Pulse Gate Multiplexer/LConn6
  Simulink-PS Converter2/RConn1 -- Six-Pulse Gate Multiplexer/LConn3
  Six-Pulse Gate Multiplexer1/RConn1 -- Gate_Signal1/RConn1
  Simulink-PS Converter9/RConn1 -- Six-Pulse Gate Multiplexer1/LConn4
  Simulink-PS Converter10/RConn1 -- Six-Pulse Gate Multiplexer1/LConn5
  Simulink-PS Converter11/RConn1 -- Six-Pulse Gate Multiplexer1/LConn6
  Simulink-PS Converter7/RConn1 -- Six-Pulse Gate Multiplexer1/LConn2
  Simulink-PS Converter8/RConn1 -- Six-Pulse Gate Multiplexer1/LConn3
  Six-Pulse Gate Multiplexer/RConn1 -- Gate_Signal/RConn1
  Simulink-PS Converter4/RConn1 -- Six-Pulse Gate Multiplexer/LConn5
  Simulink-PS Converter/RConn1 -- Six-Pulse Gate Multiplexer/LConn1
  Simulink-PS Converter3/RConn1 -- Six-Pulse Gate Multiplexer/LConn4

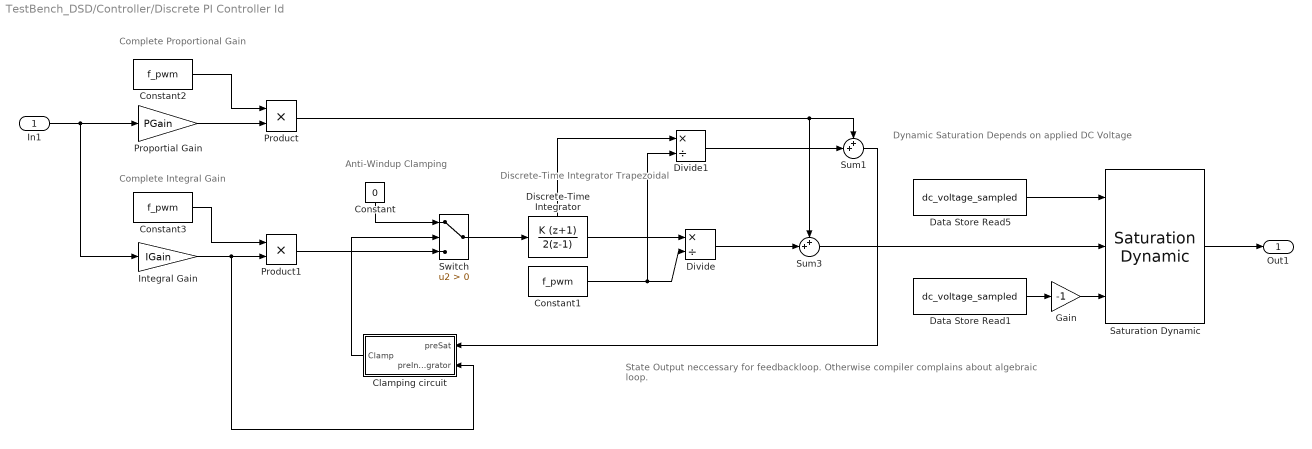
== system TestBench_DSD/Controller/Discrete PI Controller Id ==
  note: State Output neccessary for feedbackloop. Otherwise compiler complains about algebraic loop.
  note: Complete Proportional Gain
  note: Discrete-Time Integrator Trapezoidal
  note: Complete Integral Gain
  note: Anti-Windup Clamping
  note: Dynamic Saturation
      | Depends on applied DC Voltage
  In1 : Inport
  Clamping circuit : Subsystem
  Constant : Constant  DisableCoverage=on  Value=0  OutDataTypeStr=Inherit: Inherit via back propagation  PreserveConstantTs=on
  Constant1 : Constant  Value=f_pwm
  Constant2 : Constant  Value=f_pwm
  Constant3 : Constant  Value=f_pwm
  Data Store Read1 : DataStoreRead  DataStoreName=dc_voltage_sampled  IndexOptions=Index vector (dialog)  Indices=1  OutputSizes=1
  Data Store Read5 : DataStoreRead  DataStoreName=dc_voltage_sampled  IndexOptions=Index vector (dialog)  Indices=1  OutputSizes=1
  Discrete-Time Integrator : DiscreteIntegrator  IntegratorMethod=Accumulation: Trapezoidal  SampleTime=-1  ShowStatePort=on  ICPrevOutput=DiscIntNeverNeededParam  ICPrevScaledInput=DiscIntNeverNeededParam
  Divide : Product  Inputs=*/
  Divide1 : Product  Inputs=*/
  Gain : Gain  Gain=-1
  Integral Gain : Gain  Gain=IGain
  Product : Product
  Product1 : Product
  Proportial Gain : Gain  Gain=PGain
  Saturation Dynamic : simulink/Discontinuities/Saturation Dynamic  OutMin=[]  OutMax=[]  OutDataTypeStr=Inherit: Same as second input  OutDataType=fixdt(1, 16)  OutScaling=2^-10  DoSatur=off
  Sum1 : Sum  Inputs=++|
  Sum3 : Sum  Inputs=++|
  Switch : Switch  Criteria=u2 > Threshold  InputSameDT=on
  Out1 : Outport  VectorParamsAs1DForOutWhenUnconnected=off
  wires:
  Constant/1 -> Switch/1
  Clamping circuit/1(Clamp) -> Switch/2
  In1/1 -> Proportial Gain/1, Integral Gain/1
  Discrete-Time Integrator/1 -> Divide/1
  Switch/1 -> Discrete-Time Integrator/1
  Constant1/1 -> Divide/2, Divide1/2
  Sum1/1 -> Clamping circuit/1(preSat)
  Data Store Read5/1 -> Saturation Dynamic/1
  Data Store Read1/1 -> Gain/1
  Gain/1 -> Saturation Dynamic/3
  Saturation Dynamic/1 -> Out1/1
  Sum3/1 -> Saturation Dynamic/2
  Proportial Gain/1 -> Product/2
  Constant2/1 -> Product/1
  Integral Gain/1 -> Clamping circuit/2(preIntegrator), Product1/2
  Constant3/1 -> Product1/1
  Divide/1 -> Sum3/2
  Divide1/1 -> Sum1/2
  Discrete-Time Integrator/State -> Divide1/1
  Product/1 -> Sum3/1, Sum1/1
  Product1/1 -> Switch/3

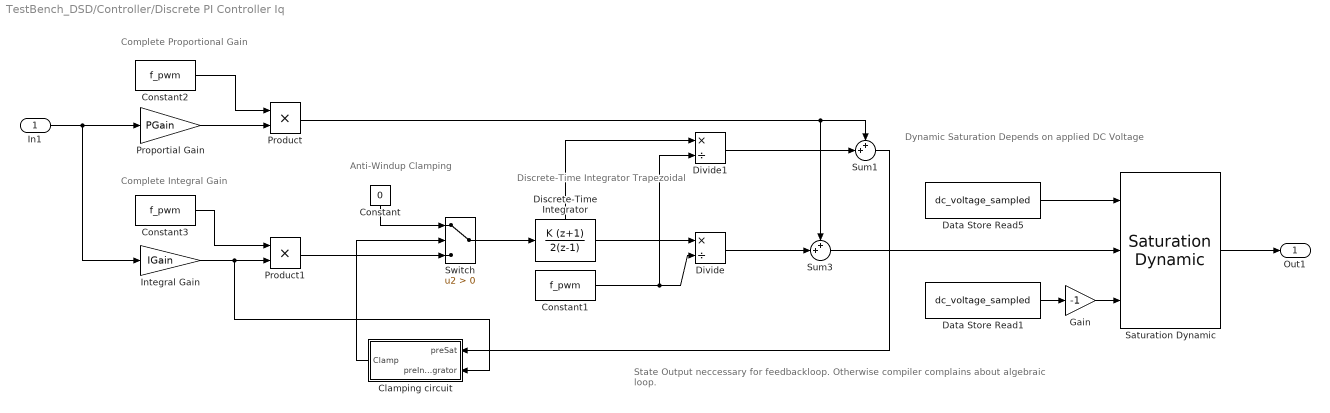
== system TestBench_DSD/Controller/Discrete PI Controller Iq ==
  note: Dynamic Saturation
      | Depends on applied DC Voltage
  note: Anti-Windup Clamping
  note: Complete Integral Gain
  note: Discrete-Time Integrator Trapezoidal
  note: Complete Proportional Gain
  note: State Output neccessary for feedbackloop. Otherwise compiler complains about algebraic loop.
  In1 : Inport
  Clamping circuit : Subsystem
  Constant : Constant  DisableCoverage=on  Value=0  OutDataTypeStr=Inherit: Inherit via back propagation  PreserveConstantTs=on
  Constant1 : Constant  Value=f_pwm
  Constant2 : Constant  Value=f_pwm
  Constant3 : Constant  Value=f_pwm
  Data Store Read1 : DataStoreRead  DataStoreName=dc_voltage_sampled  IndexOptions=Index vector (dialog)  Indices=1  OutputSizes=1
  Data Store Read5 : DataStoreRead  DataStoreName=dc_voltage_sampled  IndexOptions=Index vector (dialog)  Indices=1  OutputSizes=1
  Discrete-Time Integrator : DiscreteIntegrator  IntegratorMethod=Accumulation: Trapezoidal  SampleTime=-1  ShowStatePort=on  ICPrevOutput=DiscIntNeverNeededParam  ICPrevScaledInput=DiscIntNeverNeededParam
  Divide : Product  Inputs=*/
  Divide1 : Product  Inputs=*/
  Gain : Gain  Gain=-1
  Integral Gain : Gain  Gain=IGain
  Product : Product
  Product1 : Product
  Proportial Gain : Gain  Gain=PGain
  Saturation Dynamic : simulink/Discontinuities/Saturation Dynamic  OutMin=[]  OutMax=[]  OutDataTypeStr=Inherit: Same as second input  OutDataType=fixdt(1, 16)  OutScaling=2^-10  DoSatur=off
  Sum1 : Sum  Inputs=++|
  Sum3 : Sum  Inputs=++|
  Switch : Switch  Criteria=u2 > Threshold  InputSameDT=on
  Out1 : Outport  VectorParamsAs1DForOutWhenUnconnected=off
  wires:
  Constant3/1 -> Product1/1
  Integral Gain/1 -> Clamping circuit/2(preIntegrator), Product1/2
  Constant2/1 -> Product/1
  Proportial Gain/1 -> Product/2
  Saturation Dynamic/1 -> Out1/1
  Gain/1 -> Saturation Dynamic/3
  Data Store Read1/1 -> Gain/1
  Data Store Read5/1 -> Saturation Dynamic/1
  Sum1/1 -> Clamping circuit/1(preSat)
  Constant1/1 -> Divide1/2, Divide/2
  Switch/1 -> Discrete-Time Integrator/1
  Discrete-Time Integrator/1 -> Divide/1
  In1/1 -> Integral Gain/1, Proportial Gain/1
  Clamping circuit/1(Clamp) -> Switch/2
  Constant/1 -> Switch/1
  Divide/1 -> Sum3/2
  Discrete-Time Integrator/State -> Divide1/1
  Divide1/1 -> Sum1/2
  Sum3/1 -> Saturation Dynamic/2
  Product/1 -> Sum3/1, Sum1/1
  Product1/1 -> Switch/3

== system TestBench_DSD/Controller/Function-Call Subsystem ==
  function : TriggerPort  VariantControl=(inherit)
  Constant : Constant  Commented=on  Value=inf
  Constant1 : Constant  Commented=on
  Constant2 : Constant
  Constant7 : Constant
  Data Store Read4 : DataStoreRead  DataStoreName=Inverter  IndexOptions=Index vector (dialog)  Indices=1  OutputSizes=1
  Data Store Write : DataStoreWrite  Commented=on  DataStoreName=Sic_PhU_ChB_On  IndexOptions=Index vector (dialog)  Indices=1  OutputSizes=1
  Data Store Write1 : DataStoreWrite  Commented=on  DataStoreName=Si_PhU_ChB_On  IndexOptions=Index vector (dialog)  Indices=1  OutputSizes=1
  Data Store Write2 : DataStoreWrite  DataStoreName=Inverter  IndexOptions=Index vector (dialog)  Indices=1  OutputSizes=1
  Data Store Write6 : DataStoreWrite  DataStoreName=haltPwmSi  DataStoreElements=haltPwmSi(1)  IndexOptions=Index vector (dialog)  Indices=1  OutputSizes=1
  MATLAB Function : MATLAB Function  TreatAsAtomicUnit=on
  wires:
  Constant/1 -> Data Store Write/1
  Constant1/1 -> Data Store Write1/1
  Constant7/1 -> Data Store Write6/1
  MATLAB Function/1(y) -> Data Store Write2/1
  Data Store Read4/1 -> MATLAB Function/2(devBus)
  Constant2/1 -> MATLAB Function/1(phase)

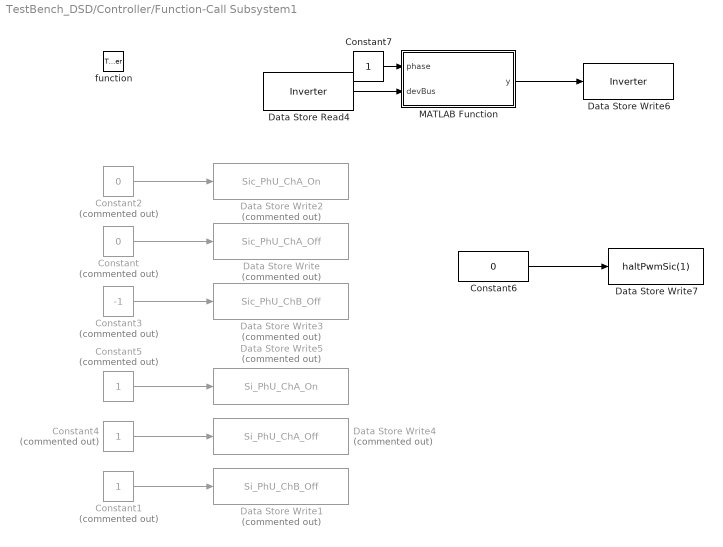
== system TestBench_DSD/Controller/Function-Call Subsystem1 ==
  function : TriggerPort  VariantControl=(inherit)
  Constant : Constant  Commented=on  Value=0
  Constant1 : Constant  Commented=on
  Constant2 : Constant  Commented=on  Value=0
  Constant3 : Constant  Commented=on  Value=-1
  Constant4 : Constant  Commented=on
  Constant5 : Constant  Commented=on
  Constant6 : Constant  Value=0
  Constant7 : Constant
  Data Store Read4 : DataStoreRead  DataStoreName=Inverter  IndexOptions=Index vector (dialog)  Indices=1  OutputSizes=1
  Data Store Write : DataStoreWrite  Commented=on  DataStoreName=Sic_PhU_ChA_Off  IndexOptions=Index vector (dialog)  Indices=1  OutputSizes=1
  Data Store Write1 : DataStoreWrite  Commented=on  DataStoreName=Si_PhU_ChB_Off  IndexOptions=Index vector (dialog)  Indices=1  OutputSizes=1
  Data Store Write2 : DataStoreWrite  Commented=on  DataStoreName=Sic_PhU_ChA_On  IndexOptions=Index vector (dialog)  Indices=1  OutputSizes=1
  Data Store Write3 : DataStoreWrite  Commented=on  DataStoreName=Sic_PhU_ChB_Off  IndexOptions=Index vector (dialog)  Indices=1  OutputSizes=1
  Data Store Write4 : DataStoreWrite  Commented=on  DataStoreName=Si_PhU_ChA_Off  IndexOptions=Index vector (dialog)  Indices=1  OutputSizes=1
  Data Store Write5 : DataStoreWrite  Commented=on  DataStoreName=Si_PhU_ChA_On  IndexOptions=Index vector (dialog)  Indices=1  OutputSizes=1
  Data Store Write6 : DataStoreWrite  DataStoreName=Inverter  IndexOptions=Index vector (dialog)  Indices=1  OutputSizes=1
  Data Store Write7 : DataStoreWrite  DataStoreName=haltPwmSic  DataStoreElements=haltPwmSic(1)  IndexOptions=Index vector (dialog)  Indices=1  OutputSizes=1
  MATLAB Function : MATLAB Function  TreatAsAtomicUnit=on
  wires:
  Constant1/1 -> Data Store Write1/1
  Constant/1 -> Data Store Write/1
  Constant2/1 -> Data Store Write2/1
  Constant3/1 -> Data Store Write3/1
  Constant4/1 -> Data Store Write4/1
  Constant5/1 -> Data Store Write5/1
  Constant6/1 -> Data Store Write7/1
  MATLAB Function/1(y) -> Data Store Write6/1
  Data Store Read4/1 -> MATLAB Function/2(devBus)
  Constant7/1 -> MATLAB Function/1(phase)

== system TestBench_DSD/Controller/Function-Call Subsystem10 ==
  function : TriggerPort  VariantControl=(inherit)
  Constant : Constant  Commented=on
  Constant1 : Constant  Commented=on  Value=1e3
  Constant2 : Constant  Value=3
  Constant6 : Constant
  Data Store Read4 : DataStoreRead  DataStoreName=Inverter  IndexOptions=Index vector (dialog)  Indices=1  OutputSizes=1
  Data Store Write : DataStoreWrite  Commented=on  DataStoreName=Sic_PhU_ChB_On  IndexOptions=Index vector (dialog)  Indices=1  OutputSizes=1
  Data Store Write1 : DataStoreWrite  Commented=on  DataStoreName=Si_PhU_ChB_On  IndexOptions=Index vector (dialog)  Indices=1  OutputSizes=1
  Data Store Write2 : DataStoreWrite  DataStoreName=Inverter  IndexOptions=Index vector (dialog)  Indices=1  OutputSizes=1
  Data Store Write7 : DataStoreWrite  DataStoreName=haltPwmSic  DataStoreElements=haltPwmSic(3)  IndexOptions=Index vector (dialog)  Indices=1  OutputSizes=1
  MATLAB Function : MATLAB Function  TreatAsAtomicUnit=on
  wires:
  Constant/1 -> Data Store Write/1
  Constant1/1 -> Data Store Write1/1
  Constant6/1 -> Data Store Write7/1
  MATLAB Function/1(y) -> Data Store Write2/1
  Data Store Read4/1 -> MATLAB Function/2(devBus)
  Constant2/1 -> MATLAB Function/1(phase)

== system TestBench_DSD/Controller/Function-Call Subsystem11 ==
  function : TriggerPort  VariantControl=(inherit)
  Constant : Constant  Commented=on
  Constant1 : Constant  Commented=on  Value=-1
  Constant2 : Constant  Commented=on
  Constant3 : Constant  Commented=on
  Constant4 : Constant  Commented=on  Value=0
  Constant5 : Constant  Commented=on  Value=0
  Constant6 : Constant  Value=3
  Constant7 : Constant  Value=0
  Data Store Read4 : DataStoreRead  DataStoreName=Inverter  IndexOptions=Index vector (dialog)  Indices=1  OutputSizes=1
  Data Store Write : DataStoreWrite  Commented=on  DataStoreName=Sic_PhU_ChA_Off  IndexOptions=Index vector (dialog)  Indices=1  OutputSizes=1
  Data Store Write1 : DataStoreWrite  Commented=on  DataStoreName=Si_PhU_ChB_Off  IndexOptions=Index vector (dialog)  Indices=1  OutputSizes=1
  Data Store Write2 : DataStoreWrite  Commented=on  DataStoreName=Sic_PhU_ChA_On  IndexOptions=Index vector (dialog)  Indices=1  OutputSizes=1
  Data Store Write3 : DataStoreWrite  Commented=on  DataStoreName=Sic_PhU_ChB_Off  IndexOptions=Index vector (dialog)  Indices=1  OutputSizes=1
  Data Store Write4 : DataStoreWrite  Commented=on  DataStoreName=Si_PhU_ChA_Off  IndexOptions=Index vector (dialog)  Indices=1  OutputSizes=1
  Data Store Write5 : DataStoreWrite  Commented=on  DataStoreName=Si_PhU_ChA_On  IndexOptions=Index vector (dialog)  Indices=1  OutputSizes=1
  Data Store Write6 : DataStoreWrite  DataStoreName=haltPwmSi  DataStoreElements=haltPwmSi(3)  IndexOptions=Index vector (dialog)  Indices=1  OutputSizes=1
  Data Store Write7 : DataStoreWrite  DataStoreName=Inverter  IndexOptions=Index vector (dialog)  Indices=1  OutputSizes=1
  MATLAB Function : MATLAB Function  TreatAsAtomicUnit=on
  wires:
  Constant1/1 -> Data Store Write1/1
  Constant/1 -> Data Store Write/1
  Constant2/1 -> Data Store Write2/1
  Constant3/1 -> Data Store Write3/1
  Constant4/1 -> Data Store Write4/1
  Constant5/1 -> Data Store Write5/1
  Constant7/1 -> Data Store Write6/1
  Data Store Read4/1 -> MATLAB Function/2(devBus)
  MATLAB Function/1(y) -> Data Store Write7/1
  Constant6/1 -> MATLAB Function/1(phase)

== system TestBench_DSD/Controller/Function-Call Subsystem2 ==
  function : TriggerPort  VariantControl=(inherit)
  Constant : Constant  Commented=on
  Constant1 : Constant  Commented=on  Value=1e3
  Constant2 : Constant
  Constant6 : Constant
  Data Store Read4 : DataStoreRead  DataStoreName=Inverter  IndexOptions=Index vector (dialog)  Indices=1  OutputSizes=1
  Data Store Write : DataStoreWrite  Commented=on  DataStoreName=Sic_PhU_ChB_On  IndexOptions=Index vector (dialog)  Indices=1  OutputSizes=1
  Data Store Write1 : DataStoreWrite  Commented=on  DataStoreName=Si_PhU_ChB_On  IndexOptions=Index vector (dialog)  Indices=1  OutputSizes=1
  Data Store Write2 : DataStoreWrite  DataStoreName=Inverter  IndexOptions=Index vector (dialog)  Indices=1  OutputSizes=1
  Data Store Write7 : DataStoreWrite  DataStoreName=haltPwmSic  DataStoreElements=haltPwmSic(1)  IndexOptions=Index vector (dialog)  Indices=1  OutputSizes=1
  MATLAB Function : MATLAB Function  TreatAsAtomicUnit=on
  wires:
  Constant/1 -> Data Store Write/1
  Constant1/1 -> Data Store Write1/1
  Constant6/1 -> Data Store Write7/1
  MATLAB Function/1(y) -> Data Store Write2/1
  Data Store Read4/1 -> MATLAB Function/2(devBus)
  Constant2/1 -> MATLAB Function/1(phase)

== system TestBench_DSD/Controller/Function-Call Subsystem3 ==
  function : TriggerPort  VariantControl=(inherit)
  Constant : Constant  Commented=on
  Constant1 : Constant  Commented=on  Value=-1
  Constant2 : Constant  Commented=on
  Constant3 : Constant  Commented=on
  Constant4 : Constant  Commented=on  Value=0
  Constant5 : Constant  Commented=on  Value=0
  Constant6 : Constant
  Constant7 : Constant  Value=0
  Data Store Read4 : DataStoreRead  DataStoreName=Inverter  IndexOptions=Index vector (dialog)  Indices=1  OutputSizes=1
  Data Store Write : DataStoreWrite  Commented=on  DataStoreName=Sic_PhU_ChA_Off  IndexOptions=Index vector (dialog)  Indices=1  OutputSizes=1
  Data Store Write1 : DataStoreWrite  Commented=on  DataStoreName=Si_PhU_ChB_Off  IndexOptions=Index vector (dialog)  Indices=1  OutputSizes=1
  Data Store Write2 : DataStoreWrite  Commented=on  DataStoreName=Sic_PhU_ChA_On  IndexOptions=Index vector (dialog)  Indices=1  OutputSizes=1
  Data Store Write3 : DataStoreWrite  Commented=on  DataStoreName=Sic_PhU_ChB_Off  IndexOptions=Index vector (dialog)  Indices=1  OutputSizes=1
  Data Store Write4 : DataStoreWrite  Commented=on  DataStoreName=Si_PhU_ChA_Off  IndexOptions=Index vector (dialog)  Indices=1  OutputSizes=1
  Data Store Write5 : DataStoreWrite  Commented=on  DataStoreName=Si_PhU_ChA_On  IndexOptions=Index vector (dialog)  Indices=1  OutputSizes=1
  Data Store Write6 : DataStoreWrite  DataStoreName=haltPwmSi  DataStoreElements=haltPwmSi(1)  IndexOptions=Index vector (dialog)  Indices=1  OutputSizes=1
  Data Store Write7 : DataStoreWrite  DataStoreName=Inverter  IndexOptions=Index vector (dialog)  Indices=1  OutputSizes=1
  MATLAB Function : MATLAB Function  TreatAsAtomicUnit=on
  wires:
  Constant1/1 -> Data Store Write1/1
  Constant/1 -> Data Store Write/1
  Constant2/1 -> Data Store Write2/1
  Constant3/1 -> Data Store Write3/1
  Constant4/1 -> Data Store Write4/1
  Constant5/1 -> Data Store Write5/1
  Constant7/1 -> Data Store Write6/1
  Data Store Read4/1 -> MATLAB Function/2(devBus)
  MATLAB Function/1(y) -> Data Store Write7/1
  Constant6/1 -> MATLAB Function/1(phase)
